simulink model "sampleModel106"  (R2022a)
settings: Solver=VariableStepAuto  StartTime=0.0  StopTime=10.0  RelTol=1e-3
undefined symbols (not defined in the file): DiscIntNeverNeededParam, magnitude, Newton, Raphson
libraries: simulink x379, slpidlib x89
(part 10 of 16)

== system sampleModel106/cfblk79/cfblk7/cfblk11/cfblk12 ==
  cfblk1 : Inport
  cfblk13 : Inport  Port=2
  cfblk14 : Inport  Port=3
  cfblk10 : Signum
  cfblk11 : Constant  Value=[417220800.929518]  SampleTime=1
  cfblk12 : Constant  Value=[-589398286.856220]  SampleTime=1
  cfblk3 : simulink/Discrete/Transfer Fcn First Order  PoleZ=0.95  ICPrevOutput=0.0  DoSatur=off
  cfblk4 : simulink/Discrete/Tapped Delay  vinit=0.0  samptime=-1  NumDelays=1  DelayOrder=Oldest  includeCurrent=off
  cfblk5 : DiscreteStateSpace
  cfblk6 : DiscreteTransferFcn  SampleTime=1
  cfblk7 : Delay  SampleTime=1
  cfblk8 : Sum  Inputs=|++
  cfblk9 : Polyval  Coefs=[ +2.081618890e-019, -1.441693666e-014, +4.719686976e-010, -8.536869453e-006, +1.621573104e-001, -8.087801117e+001 ]
  cfblk2 : Outport
  wires:
  cfblk6/1 -> cfblk5/1
  cfblk5/1 -> cfblk3/1
  cfblk3/1 -> cfblk4/1
  cfblk14/1 -> cfblk7/1
  cfblk13/1 -> cfblk9/1
  cfblk11/1 -> cfblk10/1
  cfblk10/1 -> cfblk6/1
  cfblk8/1 -> cfblk2/1
  cfblk7/1 -> cfblk8/1
  cfblk1/1 -> cfblk8/2

== system sampleModel106/cfblk79/cfblk7/cfblk11/cfblk9 ==
  cfblk1 : Inport
  cfblk11 : Inport  Port=2
  cfblk12 : Inport  Port=3
  cfblk10 : Constant  Value=[-693543349.036448]  SampleTime=1
  cfblk3 : DotProduct  OutDataTypeStr=Inherit: Inherit via internal rule
  cfblk4 : Gain  Gain=[456492011.111705]
  cfblk5 : Rounding
  cfblk6 : Squeeze
  cfblk7 : DotProduct  OutDataTypeStr=Inherit: Inherit via internal rule
  cfblk8 : Signum
  cfblk9 : Constant  Value=[-488837206.320913]  SampleTime=1
  cfblk2 : Outport
  cfblk13 : Outport  Port=2
  cfblk14 : Outport  Port=3
  wires:
  cfblk4/1 -> cfblk14/1
  cfblk5/1 -> cfblk8/1
  cfblk11/1 -> cfblk7/1
  cfblk9/1 -> cfblk5/1
  cfblk10/1 -> cfblk6/1
  cfblk3/1 -> cfblk2/1
  cfblk12/1 -> cfblk7/2
  cfblk6/1 -> cfblk3/1
  cfblk1/1 -> cfblk4/1
  cfblk7/1 -> cfblk13/1
  cfblk8/1 -> cfblk3/2

== system sampleModel106/cfblk79/cfblk7/cfblk12/cfblk11 ==
  cfblk1 : Inport
  cfblk9 : Inport  Port=2
  cfblk3 : simulink/Discrete/Transfer Fcn Real Zero  ZeroZ=0.75  ICPrevInput=0.0  DoSatur=off
      settings: SourceProductBaseCode=SL
  cfblk4 : simulink/Math Operations/MinMax Running Resettable  Function=min  vinit=0.0
  cfblk5 : Sqrt  Operator=rSqrt  AlgorithmType=Newton-Raphson
  cfblk6 : Math  Operator=hermitian
  cfblk7 : UnaryMinus
  cfblk8 : Constant  Value=[197231009.241030]  SampleTime=1
  cfblk2 : Outport
  wires:
  cfblk8/1 -> cfblk7/1
  cfblk1/1 -> cfblk6/1
  cfblk6/1 -> cfblk3/1
  cfblk4/1 -> cfblk2/1
  cfblk3/1 -> cfblk5/1
  cfblk5/1 -> cfblk4/1
  cfblk9/1 -> cfblk4/2

== system sampleModel106/cfblk79/cfblk7/cfblk12/cfblk12 ==
  cfblk1 : Inport
  cfblk10 : Polyval  Coefs=[ +2.081618890e-019, -1.441693666e-014, +4.719686976e-010, -8.536869453e-006, +1.621573104e-001, -8.087801117e+001 ]
  cfblk11 : Constant  Value=[-737910004.264372]  SampleTime=1
  cfblk12 : Constant  Value=[702082945.939267]  SampleTime=1
  cfblk13 : Constant  Value=[-981193615.725488]  SampleTime=1
  cfblk14 : Constant  Value=[-728228126.014809]  SampleTime=1
  cfblk15 : Constant  Value=[-356449572.036937]  SampleTime=1
  cfblk18 : Delay  SampleTime=1
  cfblk3 : DiscreteTransferFcn  SampleTime=1
  cfblk4 : Delay  DelayLengthSource=Input port  SampleTime=1
      settings: InputPortMap=u0,p1
  cfblk5 : UnitDelay  HasFrameUpgradeWarning=on
  cfblk6 : Product
  cfblk7 : Sqrt
  cfblk8 : Rounding
  cfblk9 : Gain  Gain=[623761261.105977]
  cfblk2 : Outport
  cfblk16 : Outport  Port=2
  cfblk17 : Outport  Port=3
  wires:
  cfblk8/1 -> cfblk10/1
  cfblk3/1 -> cfblk6/1
  cfblk15/1 -> cfblk4/1
  cfblk7/1 -> cfblk9/1
  cfblk4/1 -> cfblk16/1
  cfblk9/1 -> cfblk8/1
  cfblk14/1 -> cfblk2/1
  cfblk10/1 -> cfblk5/1
  cfblk13/1 -> cfblk6/2
  cfblk11/1 -> cfblk7/1
  cfblk1/1 -> cfblk4/2
  cfblk5/1 -> cfblk17/1
  cfblk6/1 -> cfblk18/1
  cfblk18/1 -> cfblk3/1

== system sampleModel106/cfblk79/cfblk7/cfblk12/cfblk13 ==
  cfblk1 : Inport
  cfblk10 : Inport  Port=2
  cfblk3 : DiscreteStateSpace
  cfblk4 : DiscreteIntegrator  ICPrevOutput=DiscIntNeverNeededParam  ICPrevScaledInput=DiscIntNeverNeededParam
  cfblk5 : simulink/Discrete/Transfer Fcn Real Zero  ZeroZ=0.75  ICPrevInput=0.0  DoSatur=off
      settings: SourceProductBaseCode=SL
  cfblk6 : Delay  DelayLengthSource=Input port  SampleTime=1
      settings: InputPortMap=u0,p1
  cfblk7 : Sqrt
  cfblk8 : Assignment  DiagnosticForDimensions=Warning  IndexOptions=Index vector (dialog)  Indices=1  OutputSizes=1
  cfblk9 : Sum  Inputs=+
  cfblk2 : Outport
  cfblk11 : Outport  Port=2
  cfblk12 : Outport  Port=3
  wires:
  cfblk6/1 -> cfblk11/1
  cfblk10/1 -> cfblk9/1
  cfblk8/1 -> cfblk5/1
  cfblk7/1 -> cfblk12/1, cfblk3/1, cfblk6/1
  cfblk3/1 -> cfblk8/1
  cfblk9/1 -> cfblk4/1
  cfblk1/1 -> cfblk7/1
  cfblk4/1 -> cfblk8/2, cfblk6/2
  cfblk5/1 -> cfblk2/1

== system sampleModel106/cfblk79/cfblk7/cfblk12/cfblk14 ==
  cfblk1 : Inport
  cfblk12 : Inport  Port=2
  cfblk13 : Inport  Port=3
  cfblk10 : Constant  Value=[-847782743.704588]  SampleTime=1
  cfblk11 : Constant  Value=[54410108.640307]  SampleTime=1
  cfblk17 : Delay  SampleTime=1
  cfblk3 : Product  Inputs=**
  cfblk4 : Sin  TimeSource=Use external signal  SampleTime=0
  cfblk5 : Sqrt  Operator=rSqrt  AlgorithmType=Newton-Raphson
  cfblk6 : Rounding
  cfblk7 : MinMax  Function=max
  cfblk8 : MinMax  Function=max
  cfblk9 : Sum  Inputs=+-
  cfblk2 : Outport
  cfblk14 : Outport  Port=2
  cfblk15 : Outport  Port=3
  cfblk16 : Outport  Port=4
  wires:
  cfblk12/1 -> cfblk15/1
  cfblk9/1 -> cfblk8/1
  cfblk1/1 -> cfblk2/1
  cfblk5/1 -> cfblk4/1
  cfblk10/1 -> cfblk6/1, cfblk7/1
  cfblk6/1 -> cfblk14/1
  cfblk13/1 -> cfblk5/1
  cfblk7/1 -> cfblk16/1
  cfblk4/1 -> cfblk3/1
  cfblk11/1 -> cfblk3/2
  cfblk3/1 -> cfblk9/2
  cfblk8/1 -> cfblk17/1
  cfblk17/1 -> cfblk9/1

== system sampleModel106/cfblk79/cfblk7/cfblk13/cfblk10 ==
  cfblk1 : Inport
  cfblk8 : Inport  Port=2
  cfblk9 : Inport  Port=3
  Action Port : ActionPort  ActionPortLabel=else
  cfblk10 : Delay
  cfblk3 : Delay  DelayLengthSource=Input port
      settings: InputPortMap=u0,p1
  cfblk4 : slpidlib/PID Controller  Controller=PID  Form=Parallel  TimeDomain=Discrete-time  UseExternalTs=off  SampleTime=-1  IntegratorMethod=Forward Euler  FilterMethod=Forward Euler  ControllerParametersSource=internal  P=1  I=1  UseKiTs=off  D=0  N=100  UseFilter=on  TunerSelectOption=Transfer Function Based (PID Tuner App)  InitialConditionSource=internal  InitialConditionForIntegrator=0  InitialConditionForFilter=0  DifferentiatorICPrevScaledInput=0  ExternalReset=none  TrackingMode=off  Kt=1  LimitOutput=off  SatLimitsSource=internal  UpperSaturationLimit=inf  LowerSaturationLimit=-inf  LinearizeAsGain=off  AntiWindupMode=none  Kb=1  POutMin=[]  POutMax=[]  IOutMin=[]  IOutMax=[]  DOutMin=[]  DOutMax=[]  NOutMin=[]  NOutMax=[]  SumOutMin=[]  SumOutMax=[]  SaturationOutMin=[]  SaturationOutMax=[]  PParamMin=[]  PParamMax=[]  IParamMin=[]  IParamMax=[]  DParamMin=[]  DParamMax=[]  NParamMin=[]  NParamMax=[]  KbParamMin=[]  KbParamMax=[]  KtParamMin=[]  KtParamMax=[]  KbOutMin=[]  KbOutMax=[]  KtOutMin=[]  KtOutMax=[]  IntegratorOutMin=[]  IntegratorOutMax=[]  FilterOutMin=[]  FilterOutMax=[]  SumI1OutMin=[]  SumI1OutMax=[]  SumI2OutMin=[]  SumI2OutMax=[]  SumI3OutMin=[]  SumI3OutMax=[]  SumI4OutMin=[]  SumI4OutMax=[]  SumDOutMin=[]  SumDOutMax=[]  DifferentiatorOutMin=[]  DifferentiatorOutMax=[]  FilterDiffOutCoefMin=[]  FilterDiffOutCoefMax=[]  ReciprocalOutMin=[]  ReciprocalOutMax=[]  SumDenOutMin=[]  SumDenOutMax=[]  SumNumOutMin=[]  SumNumOutMax=[]  DivideOutMin=[]  DivideOutMax=[]  UdiffTsProdOutMin=[]  UdiffTsProdOutMax=[]  NTsProdOutMin=[]  NTsProdOutMax=[]  UintegralTsProdOutMin=[]  UintegralTsProdOutMax=[]  UngainTsProdOutMin=[]  UngainTsProdOutMax=[]  IntegratorContinuousStateAttributes=''  IntegratorStateMustResolveToSignalObject=off  IntegratorRTWStateStorageClass=Auto  FilterContinuousStateAttributes=''  FilterStateMustResolveToSignalObject=off  FilterRTWStateStorageClass=Auto  ParallelPVariant=InternalParameters  IdealPVariant=Disabled  IVariant=InternalParameters  DVariant=InternalParameters  IntegratorVariant=Discrete  SatVariant=Disabled  AWVariant=Passthrough  PCopyVariant=Disabled  TRVariant=Disabled  FdbkBlocksVariant=Forward  IdealPFdbkVariant=Disabled  SatFdbkVariant=Disabled  DerivativeFilterVariant=ForwardEulerFilter  NVariant=InternalParameters  NCopyVariant=Disabled  FilterICVariant=InternalICsFilter  IntegratorICVariant=InternalICs  ExternalResetVariant=Disabled  TRSumVariant=Passthrough  SumFdbkVariant=Disabled  SumVariant=Sum_PID  TsampFilterVariant=InternalTs  TsampNgainVariant=Passthrough  TsampIntegralVariant=Passthrough  ExternalSaturationOutDataTypeStr=Inherit: Same as second input  aMode=0
  cfblk5 : Product  Inputs=*
  cfblk6 : PermuteDimensions
  cfblk7 : Sum  Inputs=|++
  cfblk2 : Outport
  wires:
  cfblk8/1 -> cfblk6/1
  cfblk3/1 -> cfblk7/2
  cfblk7/1 -> cfblk5/1
  cfblk9/1 -> cfblk3/1
  cfblk5/1 -> cfblk4/1
  cfblk1/1 -> cfblk3/2
  cfblk6/1 -> cfblk2/1
  cfblk4/1 -> cfblk10/1
  cfblk10/1 -> cfblk7/1

== system sampleModel106/cfblk79/cfblk7/cfblk13/cfblk6 ==
  cfblk1 : Inport
  cfblk6 : Inport  Port=2
  cfblk3 : DiscreteZeroPole  Poles=[0 0.5]  Gain=1
  cfblk4 : simulink/Math Operations/MinMax Running Resettable  Function=min  vinit=0.0
  cfblk5 : Constant  Value=[107048093.151828]  SampleTime=1
  cfblk2 : Outport
  cfblk7 : Outport  Port=2
  wires:
  cfblk5/1 -> cfblk4/1
  cfblk6/1 -> cfblk4/2
  cfblk4/1 -> cfblk7/1, cfblk3/1
  cfblk1/1 -> cfblk2/1

== system sampleModel106/cfblk79/cfblk7/cfblk13/cfblk7 ==
  cfblk1 : Inport
  cfblk11 : Inport  Port=2
  cfblk10 : Constant  Value=[433998706.675589]  SampleTime=1
  cfblk3 : simulink/Discrete/Transfer Fcn First Order  PoleZ=0.95  ICPrevOutput=0.0  DoSatur=off
  cfblk4 : PermuteDimensions
  cfblk5 : Bias  Bias=[753493053.405927]  SaturateOnIntegerOverflow=off
  cfblk6 : Sum  Inputs=+-
  cfblk7 : Sum  Inputs=+
  cfblk8 : Bias  Bias=[552868234.921718]  SaturateOnIntegerOverflow=off
  cfblk9 : Rounding
  cfblk2 : Outport
  cfblk12 : Outport  Port=2
  cfblk13 : Outport  Port=3
  cfblk14 : Outport  Port=4
  wires:
  cfblk1/1 -> cfblk3/1
  cfblk4/1 -> cfblk8/1, cfblk7/1
  cfblk10/1 -> cfblk12/1
  cfblk9/1 -> cfblk13/1, cfblk4/1
  cfblk8/1 -> cfblk2/1
  cfblk11/1 -> cfblk9/1
  cfblk3/1 -> cfblk6/1
  cfblk6/1 -> cfblk14/1
  cfblk7/1 -> cfblk5/1
  cfblk5/1 -> cfblk6/2

== system sampleModel106/cfblk79/cfblk7/cfblk13/cfblk9 ==
  cfblk1 : Inport
  cfblk13 : Inport  Port=2
  Action Port : ActionPort  ActionPortLabel=if(u1 >= 0)
  cfblk10 : Squeeze
  cfblk11 : Constant  Value=[917711784.016903]  SampleTime=1
  cfblk12 : Constant  Value=[-45160633.184772]  SampleTime=1
  cfblk3 : slpidlib/PID Controller  Controller=PID  Form=Parallel  TimeDomain=Discrete-time  UseExternalTs=off  SampleTime=-1  IntegratorMethod=Forward Euler  FilterMethod=Forward Euler  ControllerParametersSource=internal  P=1  I=1  UseKiTs=off  D=0  N=100  UseFilter=on  TunerSelectOption=Transfer Function Based (PID Tuner App)  InitialConditionSource=internal  InitialConditionForIntegrator=0  InitialConditionForFilter=0  DifferentiatorICPrevScaledInput=0  ExternalReset=none  TrackingMode=off  Kt=1  LimitOutput=off  SatLimitsSource=internal  UpperSaturationLimit=inf  LowerSaturationLimit=-inf  LinearizeAsGain=off  AntiWindupMode=none  Kb=1  POutMin=[]  POutMax=[]  IOutMin=[]  IOutMax=[]  DOutMin=[]  DOutMax=[]  NOutMin=[]  NOutMax=[]  SumOutMin=[]  SumOutMax=[]  SaturationOutMin=[]  SaturationOutMax=[]  PParamMin=[]  PParamMax=[]  IParamMin=[]  IParamMax=[]  DParamMin=[]  DParamMax=[]  NParamMin=[]  NParamMax=[]  KbParamMin=[]  KbParamMax=[]  KtParamMin=[]  KtParamMax=[]  KbOutMin=[]  KbOutMax=[]  KtOutMin=[]  KtOutMax=[]  IntegratorOutMin=[]  IntegratorOutMax=[]  FilterOutMin=[]  FilterOutMax=[]  SumI1OutMin=[]  SumI1OutMax=[]  SumI2OutMin=[]  SumI2OutMax=[]  SumI3OutMin=[]  SumI3OutMax=[]  SumI4OutMin=[]  SumI4OutMax=[]  SumDOutMin=[]  SumDOutMax=[]  DifferentiatorOutMin=[]  DifferentiatorOutMax=[]  FilterDiffOutCoefMin=[]  FilterDiffOutCoefMax=[]  ReciprocalOutMin=[]  ReciprocalOutMax=[]  SumDenOutMin=[]  SumDenOutMax=[]  SumNumOutMin=[]  SumNumOutMax=[]  DivideOutMin=[]  DivideOutMax=[]  UdiffTsProdOutMin=[]  UdiffTsProdOutMax=[]  NTsProdOutMin=[]  NTsProdOutMax=[]  UintegralTsProdOutMin=[]  UintegralTsProdOutMax=[]  UngainTsProdOutMin=[]  UngainTsProdOutMax=[]  IntegratorContinuousStateAttributes=''  IntegratorStateMustResolveToSignalObject=off  IntegratorRTWStateStorageClass=Auto  FilterContinuousStateAttributes=''  FilterStateMustResolveToSignalObject=off  FilterRTWStateStorageClass=Auto  ParallelPVariant=InternalParameters  IdealPVariant=Disabled  IVariant=InternalParameters  DVariant=InternalParameters  IntegratorVariant=Discrete  SatVariant=Disabled  AWVariant=Passthrough  PCopyVariant=Disabled  TRVariant=Disabled  FdbkBlocksVariant=Forward  IdealPFdbkVariant=Disabled  SatFdbkVariant=Disabled  DerivativeFilterVariant=ForwardEulerFilter  NVariant=InternalParameters  NCopyVariant=Disabled  FilterICVariant=InternalICsFilter  IntegratorICVariant=InternalICs  ExternalResetVariant=Disabled  TRSumVariant=Passthrough  SumFdbkVariant=Disabled  SumVariant=Sum_PID  TsampFilterVariant=InternalTs  TsampNgainVariant=Passthrough  TsampIntegralVariant=Passthrough  ExternalSaturationOutDataTypeStr=Inherit: Same as second input  aMode=0
  cfblk4 : Assignment  DiagnosticForDimensions=Warning  IndexOptions=Index vector (dialog)  Indices=1  OutputSizes=1
  cfblk5 : Signum
  cfblk6 : Squeeze
  cfblk7 : Squeeze
  cfblk8 : Reshape
  cfblk9 : Sum  Inputs=+-
  cfblk2 : Outport
  cfblk14 : Outport  Port=2
  cfblk15 : Outport  Port=3
  wires:
  cfblk6/1 -> cfblk7/1
  cfblk9/1 -> cfblk2/1
  cfblk7/1 -> cfblk15/1
  cfblk3/1 -> cfblk5/1
  cfblk5/1 -> cfblk8/1
  cfblk8/1 -> cfblk4/1
  cfblk12/1 -> cfblk14/1
  cfblk4/1 -> cfblk6/1, cfblk9/2
  cfblk13/1 -> cfblk10/1
  cfblk1/1 -> cfblk3/1
  cfblk10/1 -> cfblk9/1
  cfblk11/1 -> cfblk4/2

== system sampleModel106/cfblk79/cfblk8/cfblk10/cfblk7 ==
  cfblk1 : Inport
  cfblk6 : Inport  Port=2
  cfblk7 : Inport  Port=3
  cfblk8 : Inport  Port=4
  cfblk9 : Inport  Port=5
  cfblk3 : Delay  DelayLengthSource=Input port  SampleTime=1
      settings: InputPortMap=u0,p1
  cfblk4 : Reshape
  cfblk5 : Constant  Value=[890064737.840276]  SampleTime=1
  cfblk2 : Outport
  wires:
  cfblk9/1 -> cfblk2/1
  cfblk4/1 -> cfblk3/1
  cfblk5/1 -> cfblk3/2
  cfblk8/1 -> cfblk4/1

== system sampleModel106/cfblk79/cfblk8/cfblk10/cfblk8 ==
  cfblk1 : Inport
  cfblk9 : Inport  Port=2
  cfblk10 : Inport  Port=3
  cfblk11 : Inport  Port=4
  cfblk12 : Inport  Port=5
  cfblk3 : DiscreteTransferFcn  SampleTime=1
  cfblk4 : Rounding
  cfblk5 : Sqrt
  cfblk6 : Constant  Value=[743549077.213179]  SampleTime=1
  cfblk7 : Constant  Value=[509884695.187006]  SampleTime=1
  cfblk8 : Constant  Value=[233910695.868611]  SampleTime=1
  cfblk2 : Outport
  cfblk13 : Outport  Port=2
  cfblk14 : Outport  Port=3
  wires:
  cfblk11/1 -> cfblk4/1
  cfblk1/1 -> cfblk5/1
  cfblk10/1 -> cfblk14/1
  cfblk8/1 -> cfblk2/1
  cfblk5/1 -> cfblk13/1
  cfblk12/1 -> cfblk3/1

== system sampleModel106/cfblk79/cfblk8/cfblk11/cfblk11 ==
  cfblk1 : Inport
  cfblk12 : Inport  Port=2
  cfblk13 : Inport  Port=3
  cfblk14 : Inport  Port=4
  cfblk15 : Inport  Port=5
  cfblk16 : Inport  Port=6
  cfblk10 : Constant  Value=[847867701.646288]  SampleTime=1
  cfblk11 : Constant  Value=[-637143935.125896]  SampleTime=1
  cfblk3 : Delay  DelayLengthSource=Input port  SampleTime=1
      settings: InputPortMap=u0,p1
  cfblk4 : Polyval  Coefs=[ +2.081618890e-019, -1.441693666e-014, +4.719686976e-010, -8.536869453e-006, +1.621573104e-001, -8.087801117e+001 ]
  cfblk5 : Sum  Inputs=+
  cfblk6 : Trigonometry
  cfblk7 : Sin  TimeSource=Use external signal  SampleTime=0
  cfblk8 : Bias  Bias=[425461441.150961]  SaturateOnIntegerOverflow=off
  cfblk9 : simulink/Math Operations/MinMax Running Resettable  Function=min  vinit=0.0
  cfblk2 : Outport
  wires:
  cfblk14/1 -> cfblk7/1
  cfblk10/1 -> cfblk8/1
  cfblk16/1 -> cfblk6/1
  cfblk4/1 -> cfblk9/1
  cfblk7/1 -> cfblk4/1
  cfblk1/1 -> cfblk9/2
  cfblk5/1 -> cfblk2/1
  cfblk6/1 -> cfblk3/1
  cfblk13/1 -> cfblk3/2
  cfblk8/1 -> cfblk5/1

== system sampleModel106/cfblk79/cfblk8/cfblk11/cfblk12 ==
  cfblk1 : Inport
  cfblk9 : Inport  Port=2
  cfblk12 : Delay  SampleTime=1
  cfblk3 : simulink/Discrete/Transfer Fcn Real Zero  ZeroZ=0.75  ICPrevInput=0.0  DoSatur=off
      settings: SourceProductBaseCode=SL
  cfblk4 : UnitDelay  HasFrameUpgradeWarning=on
  cfblk5 : Rounding
  cfblk6 : Sum  Inputs=+-
  cfblk7 : DotProduct  OutDataTypeStr=Inherit: Inherit via internal rule
  cfblk8 : Constant  Value=[74573973.878207]  SampleTime=1
  cfblk2 : Outport
  cfblk10 : Outport  Port=2
  cfblk11 : Outport  Port=3
  wires:
  cfblk5/1 -> cfblk4/1
  cfblk8/1 -> cfblk11/1
  cfblk4/1 -> cfblk7/1
  cfblk6/1 -> cfblk7/2, cfblk12/1
  cfblk1/1 -> cfblk2/1
  cfblk7/1 -> cfblk10/1
  cfblk3/1 -> cfblk5/1, cfblk6/2
  cfblk9/1 -> cfblk6/1
  cfblk12/1 -> cfblk3/1

== system sampleModel106/cfblk79/cfblk8/cfblk11/cfblk18 ==
  cfblk1 : Inport
  cfblk8 : Inport  Port=2
  Action Port : ActionPort  ActionPortLabel=if(u1 >= 0)
  cfblk3 : simulink/Discrete/Transfer Fcn First Order  PoleZ=0.95  ICPrevOutput=0.0  DoSatur=off
  cfblk4 : UnitDelay  SampleTime=-1  HasFrameUpgradeWarning=on
  cfblk5 : Delay
  cfblk6 : Constant  Value=[961105.655787]  SampleTime=1
  cfblk7 : Constant  Value=[134183387.324209]  SampleTime=1
  cfblk2 : Outport
  wires:
  cfblk4/1 -> cfblk2/1
  cfblk7/1 -> cfblk4/1
  cfblk5/1 -> cfblk3/1
  cfblk6/1 -> cfblk5/1

== system sampleModel106/cfblk79/cfblk8/cfblk11/cfblk19 ==
  cfblk1 : Inport
  cfblk11 : Inport  Port=2
  cfblk12 : Inport  Port=3
  Action Port : ActionPort  ActionPortLabel=else
  cfblk10 : Sqrt
  cfblk16 : Delay
  cfblk3 : DiscreteFilter
  cfblk4 : DiscreteFir
  cfblk5 : Sum  Inputs=+-
  cfblk6 : Sum  Inputs=+-
  cfblk7 : Bias  Bias=[-421978992.975569]  SaturateOnIntegerOverflow=off
  cfblk8 : Squeeze
  cfblk9 : Product  Inputs=*
  cfblk2 : Outport
  cfblk13 : Outport  Port=2
  cfblk14 : Outport  Port=3
  cfblk15 : Outport  Port=4
  wires:
  cfblk11/1 -> cfblk8/1
  cfblk4/1 -> cfblk2/1, cfblk14/1
  cfblk5/1 -> cfblk7/1
  cfblk9/1 -> cfblk6/2
  cfblk6/1 -> cfblk10/1, cfblk5/2
  cfblk12/1 -> cfblk5/1
  cfblk3/1 -> cfblk4/1, cfblk15/1
  cfblk10/1 -> cfblk13/1
  cfblk1/1 -> cfblk9/1
  cfblk8/1 -> cfblk3/1
  cfblk7/1 -> cfblk16/1
  cfblk16/1 -> cfblk6/1

== system sampleModel106/cfblk79/cfblk8/cfblk9/cfblk9 ==
  cfblk1 : Inport
  cfblk7 : Inport  Port=2
  cfblk8 : Inport  Port=3
  cfblk9 : Inport  Port=4
  cfblk3 : DiscreteStateSpace
  cfblk4 : Polyval  Coefs=[ +2.081618890e-019, -1.441693666e-014, +4.719686976e-010, -8.536869453e-006, +1.621573104e-001, -8.087801117e+001 ]
  cfblk5 : Reshape
  cfblk6 : Constant  Value=[572215483.203508]  SampleTime=1
  cfblk2 : Outport
  cfblk10 : Outport  Port=2
  cfblk11 : Outport  Port=3
  wires:
  cfblk8/1 -> cfblk4/1
  cfblk7/1 -> cfblk2/1
  cfblk1/1 -> cfblk3/1
  cfblk5/1 -> cfblk11/1
  cfblk4/1 -> cfblk10/1
  cfblk3/1 -> cfblk5/1

== system sampleModel106/cfblk80/cfblk10/cfblk10/cfblk10 ==
  cfblk1 : Inport
  cfblk6 : Inport  Port=2
  cfblk3 : DiscreteIntegrator  ICPrevOutput=DiscIntNeverNeededParam  ICPrevScaledInput=DiscIntNeverNeededParam
  cfblk4 : simulink/Discrete/Transfer Fcn First Order  PoleZ=0.95  ICPrevOutput=0.0  DoSatur=off
  cfblk5 : simulink/Math Operations/Slider Gain  gain=1  low=0  high=2
  cfblk2 : Outport
  cfblk7 : Outport  Port=2
  wires:
  cfblk1/1 -> cfblk5/1
  cfblk4/1 -> cfblk7/1
  cfblk6/1 -> cfblk4/1
  cfblk5/1 -> cfblk3/1
  cfblk3/1 -> cfblk2/1

== system sampleModel106/cfblk80/cfblk10/cfblk10/cfblk11 ==
  cfblk1 : Inport
  cfblk9 : Inport  Port=2
  cfblk10 : Delay  SampleTime=1
  cfblk3 : Sum  Inputs=--
  cfblk4 : Sqrt  Operator=rSqrt  AlgorithmType=Newton-Raphson
  cfblk5 : simulink/Math Operations/Slider Gain  gain=1  low=0  high=2
  cfblk6 : Constant  Value=[387218485.302088]  SampleTime=1
  cfblk7 : Constant  Value=[-419599135.660851]  SampleTime=1
  cfblk8 : Constant  Value=[-709917624.129009]  SampleTime=1
  cfblk2 : Outport
  wires:
  cfblk3/1 -> cfblk4/1
  cfblk7/1 -> cfblk2/1
  cfblk9/1 -> cfblk3/2
  cfblk8/1 -> cfblk5/1
  cfblk4/1 -> cfblk10/1
  cfblk10/1 -> cfblk3/1

== system sampleModel106/cfblk80/cfblk10/cfblk10/cfblk12 ==
  cfblk1 : Inport
  cfblk6 : Inport  Port=2
  cfblk7 : Inport  Port=3
  cfblk8 : Inport  Port=4
  cfblk3 : DiscreteStateSpace
  cfblk4 : ComplexToMagnitudeAngle
  cfblk5 : Constant  Value=[132792448.593113]  SampleTime=1
  cfblk2 : Outport
  cfblk9 : Outport  Port=2
  wires:
  cfblk5/1 -> cfblk2/1
  cfblk7/1 -> cfblk3/1
  cfblk4/1 -> cfblk9/1
  cfblk1/1 -> cfblk4/1

== system sampleModel106/cfblk80/cfblk10/cfblk10/cfblk9 ==
  cfblk1 : Inport
  cfblk12 : Inport  Port=2
  cfblk13 : Inport  Port=3
  cfblk10 : Constant  Value=[69698120.127665]  SampleTime=1
  cfblk11 : Constant  Value=[-849367431.639594]  SampleTime=1
  cfblk3 : slpidlib/PID Controller  Controller=PID  Form=Parallel  TimeDomain=Discrete-time  UseExternalTs=off  SampleTime=1  IntegratorMethod=Forward Euler  FilterMethod=Forward Euler  ControllerParametersSource=internal  P=1  I=1  UseKiTs=off  D=0  N=100  UseFilter=on  TunerSelectOption=Transfer Function Based (PID Tuner App)  InitialConditionSource=internal  InitialConditionForIntegrator=0  InitialConditionForFilter=0  DifferentiatorICPrevScaledInput=0  ExternalReset=none  TrackingMode=off  Kt=1  LimitOutput=off  SatLimitsSource=internal  UpperSaturationLimit=inf  LowerSaturationLimit=-inf  LinearizeAsGain=off  AntiWindupMode=none  Kb=1  POutMin=[]  POutMax=[]  IOutMin=[]  IOutMax=[]  DOutMin=[]  DOutMax=[]  NOutMin=[]  NOutMax=[]  SumOutMin=[]  SumOutMax=[]  SaturationOutMin=[]  SaturationOutMax=[]  PParamMin=[]  PParamMax=[]  IParamMin=[]  IParamMax=[]  DParamMin=[]  DParamMax=[]  NParamMin=[]  NParamMax=[]  KbParamMin=[]  KbParamMax=[]  KtParamMin=[]  KtParamMax=[]  KbOutMin=[]  KbOutMax=[]  KtOutMin=[]  KtOutMax=[]  IntegratorOutMin=[]  IntegratorOutMax=[]  FilterOutMin=[]  FilterOutMax=[]  SumI1OutMin=[]  SumI1OutMax=[]  SumI2OutMin=[]  SumI2OutMax=[]  SumI3OutMin=[]  SumI3OutMax=[]  SumI4OutMin=[]  SumI4OutMax=[]  SumDOutMin=[]  SumDOutMax=[]  DifferentiatorOutMin=[]  DifferentiatorOutMax=[]  FilterDiffOutCoefMin=[]  FilterDiffOutCoefMax=[]  ReciprocalOutMin=[]  ReciprocalOutMax=[]  SumDenOutMin=[]  SumDenOutMax=[]  SumNumOutMin=[]  SumNumOutMax=[]  DivideOutMin=[]  DivideOutMax=[]  UdiffTsProdOutMin=[]  UdiffTsProdOutMax=[]  NTsProdOutMin=[]  NTsProdOutMax=[]  UintegralTsProdOutMin=[]  UintegralTsProdOutMax=[]  UngainTsProdOutMin=[]  UngainTsProdOutMax=[]  IntegratorContinuousStateAttributes=''  IntegratorStateMustResolveToSignalObject=off  IntegratorRTWStateStorageClass=Auto  FilterContinuousStateAttributes=''  FilterStateMustResolveToSignalObject=off  FilterRTWStateStorageClass=Auto  ParallelPVariant=InternalParameters  IdealPVariant=Disabled  IVariant=InternalParameters  DVariant=InternalParameters  IntegratorVariant=Discrete  SatVariant=Disabled  AWVariant=Passthrough  PCopyVariant=Disabled  TRVariant=Disabled  FdbkBlocksVariant=Forward  IdealPFdbkVariant=Disabled  SatFdbkVariant=Disabled  DerivativeFilterVariant=ForwardEulerFilter  NVariant=InternalParameters  NCopyVariant=Disabled  FilterICVariant=InternalICsFilter  IntegratorICVariant=InternalICs  ExternalResetVariant=Disabled  TRSumVariant=Passthrough  SumFdbkVariant=Disabled  SumVariant=Sum_PID  TsampFilterVariant=InternalTs  TsampNgainVariant=Passthrough  TsampIntegralVariant=Passthrough  ExternalSaturationOutDataTypeStr=Inherit: Same as second input  aMode=0
  cfblk4 : simulink/Discrete/Transfer Fcn First Order  PoleZ=0.95  ICPrevOutput=0.0  DoSatur=off
  cfblk5 : DiscreteFir  SampleTime=1
  cfblk6 : Product
  cfblk7 : Sin  TimeSource=Use external signal  SampleTime=0
  cfblk8 : Gain  Gain=[-430636425.139552]
  cfblk9 : Constant  Value=[941054476.673307]  SampleTime=1
  cfblk2 : Outport
  wires:
  cfblk4/1 -> cfblk5/1
  cfblk10/1 -> cfblk2/1
  cfblk9/1 -> cfblk6/1
  cfblk7/1 -> cfblk4/1
  cfblk6/1 -> cfblk8/1
  cfblk5/1 -> cfblk3/1
  cfblk13/1 -> cfblk6/2
  cfblk8/1 -> cfblk7/1

== system sampleModel106/cfblk80/cfblk10/cfblk11/cfblk10 ==
  cfblk1 : Inport
  cfblk10 : Inport  Port=2
  cfblk3 : slpidlib/PID Controller  Controller=PID  Form=Parallel  TimeDomain=Discrete-time  UseExternalTs=off  SampleTime=1  IntegratorMethod=Forward Euler  FilterMethod=Forward Euler  ControllerParametersSource=internal  P=1  I=1  UseKiTs=off  D=0  N=100  UseFilter=on  TunerSelectOption=Transfer Function Based (PID Tuner App)  InitialConditionSource=internal  InitialConditionForIntegrator=0  InitialConditionForFilter=0  DifferentiatorICPrevScaledInput=0  ExternalReset=none  TrackingMode=off  Kt=1  LimitOutput=off  SatLimitsSource=internal  UpperSaturationLimit=inf  LowerSaturationLimit=-inf  LinearizeAsGain=off  AntiWindupMode=none  Kb=1  POutMin=[]  POutMax=[]  IOutMin=[]  IOutMax=[]  DOutMin=[]  DOutMax=[]  NOutMin=[]  NOutMax=[]  SumOutMin=[]  SumOutMax=[]  SaturationOutMin=[]  SaturationOutMax=[]  PParamMin=[]  PParamMax=[]  IParamMin=[]  IParamMax=[]  DParamMin=[]  DParamMax=[]  NParamMin=[]  NParamMax=[]  KbParamMin=[]  KbParamMax=[]  KtParamMin=[]  KtParamMax=[]  KbOutMin=[]  KbOutMax=[]  KtOutMin=[]  KtOutMax=[]  IntegratorOutMin=[]  IntegratorOutMax=[]  FilterOutMin=[]  FilterOutMax=[]  SumI1OutMin=[]  SumI1OutMax=[]  SumI2OutMin=[]  SumI2OutMax=[]  SumI3OutMin=[]  SumI3OutMax=[]  SumI4OutMin=[]  SumI4OutMax=[]  SumDOutMin=[]  SumDOutMax=[]  DifferentiatorOutMin=[]  DifferentiatorOutMax=[]  FilterDiffOutCoefMin=[]  FilterDiffOutCoefMax=[]  ReciprocalOutMin=[]  ReciprocalOutMax=[]  SumDenOutMin=[]  SumDenOutMax=[]  SumNumOutMin=[]  SumNumOutMax=[]  DivideOutMin=[]  DivideOutMax=[]  UdiffTsProdOutMin=[]  UdiffTsProdOutMax=[]  NTsProdOutMin=[]  NTsProdOutMax=[]  UintegralTsProdOutMin=[]  UintegralTsProdOutMax=[]  UngainTsProdOutMin=[]  UngainTsProdOutMax=[]  IntegratorContinuousStateAttributes=''  IntegratorStateMustResolveToSignalObject=off  IntegratorRTWStateStorageClass=Auto  FilterContinuousStateAttributes=''  FilterStateMustResolveToSignalObject=off  FilterRTWStateStorageClass=Auto  ParallelPVariant=InternalParameters  IdealPVariant=Disabled  IVariant=InternalParameters  DVariant=InternalParameters  IntegratorVariant=Discrete  SatVariant=Disabled  AWVariant=Passthrough  PCopyVariant=Disabled  TRVariant=Disabled  FdbkBlocksVariant=Forward  IdealPFdbkVariant=Disabled  SatFdbkVariant=Disabled  DerivativeFilterVariant=ForwardEulerFilter  NVariant=InternalParameters  NCopyVariant=Disabled  FilterICVariant=InternalICsFilter  IntegratorICVariant=InternalICs  ExternalResetVariant=Disabled  TRSumVariant=Passthrough  SumFdbkVariant=Disabled  SumVariant=Sum_PID  TsampFilterVariant=InternalTs  TsampNgainVariant=Passthrough  TsampIntegralVariant=Passthrough  ExternalSaturationOutDataTypeStr=Inherit: Same as second input  aMode=0
  cfblk4 : DiscreteZeroPole  Poles=[0 0.5]  Gain=1
  cfblk5 : simulink/Discrete/Difference  ICPrevInput=0.0  OutMin=[]  OutMax=[]  OutDataTypeStr=Inherit: Inherit via back propagation  OutDataType=fixdt(1, 16)  OutScaling=2^-10  DoSatur=off
  cfblk6 : Product  Inputs=**
  cfblk7 : Sqrt  Operator=rSqrt  AlgorithmType=Newton-Raphson
  cfblk8 : Constant  Value=[-878471034.084976]  SampleTime=1
  cfblk9 : Constant  Value=[980508287.317108]  SampleTime=1
  cfblk2 : Outport
  cfblk11 : Outport  Port=2
  cfblk12 : Outport  Port=3
  wires:
  cfblk1/1 -> cfblk3/1
  cfblk5/1 -> cfblk4/1
  cfblk4/1 -> cfblk7/1
  cfblk9/1 -> cfblk11/1
  cfblk3/1 -> cfblk2/1
  cfblk8/1 -> cfblk12/1
  cfblk7/1 -> cfblk6/1
  cfblk10/1 -> cfblk5/1, cfblk6/2

== system sampleModel106/cfblk80/cfblk10/cfblk11/cfblk11 ==
  cfblk1 : Inport
  cfblk9 : Inport  Port=2
  cfblk10 : Delay  SampleTime=1
  cfblk3 : DiscreteStateSpace
  cfblk4 : DiscreteIntegrator  ICPrevOutput=DiscIntNeverNeededParam  ICPrevScaledInput=DiscIntNeverNeededParam
  cfblk5 : simulink/Math Operations/Slider Gain  gain=1  low=0  high=2
  cfblk6 : Rounding
  cfblk7 : UnaryMinus
  cfblk8 : Constant  Value=[833066314.757185]  SampleTime=1
  cfblk2 : Outport
  wires:
  cfblk3/1 -> cfblk7/1
  cfblk4/1 -> cfblk5/1
  cfblk9/1 -> cfblk2/1
  cfblk7/1 -> cfblk6/1
  cfblk8/1 -> cfblk3/1
  cfblk5/1 -> cfblk10/1
  cfblk10/1 -> cfblk4/1

== system sampleModel106/cfblk80/cfblk10/cfblk11/cfblk12 ==
  cfblk1 : Inport
  cfblk10 : Inport  Port=2
  cfblk11 : Inport  Port=3
  cfblk12 : Inport  Port=4
  cfblk3 : Product
  cfblk4 : Product  Inputs=*
  cfblk5 : Gain  Gain=[-892362151.792230]
  cfblk6 : Signum
  cfblk7 : Constant  Value=[-936145302.178599]  SampleTime=1
  cfblk8 : Constant  Value=[-860922800.001276]  SampleTime=1
  cfblk9 : Constant  Value=[-857530112.678363]  SampleTime=1
  cfblk2 : Outport
  cfblk13 : Outport  Port=2
  wires:
  cfblk7/1 -> cfblk5/1
  cfblk8/1 -> cfblk6/1
  cfblk4/1 -> cfblk2/1
  cfblk11/1 -> cfblk13/1
  cfblk10/1 -> cfblk3/1
  cfblk9/1 -> cfblk3/2
  cfblk6/1 -> cfblk4/1

== system sampleModel106/cfblk80/cfblk10/cfblk11/cfblk13 ==
  cfblk1 : Inport
  cfblk6 : Inport  Port=2
  cfblk7 : Inport  Port=3
  cfblk8 : Inport  Port=4
  cfblk3 : Sum  Inputs=+-
  cfblk4 : Product  Inputs=**
  cfblk5 : Polyval  Coefs=[ +2.081618890e-019, -1.441693666e-014, +4.719686976e-010, -8.536869453e-006, +1.621573104e-001, -8.087801117e+001 ]
  cfblk2 : Outport
  cfblk9 : Outport  Port=2
  cfblk10 : Outport  Port=3
  cfblk11 : Outport  Port=4
  cfblk12 : Outport  Port=5
  wires:
  cfblk6/1 -> cfblk9/1
  cfblk1/1 -> cfblk11/1
  cfblk4/1 -> cfblk2/1, cfblk3/2
  cfblk7/1 -> cfblk4/1
  cfblk5/1 -> cfblk4/2
  cfblk8/1 -> cfblk5/1, cfblk3/1
  cfblk3/1 -> cfblk12/1, cfblk10/1

== system sampleModel106/cfblk80/cfblk10/cfblk11/cfblk16 ==
  cfblk1 : Inport
  cfblk13 : Inport  Port=2
  Action Port : ActionPort  ActionPortLabel=if(u1 >= 0)
  cfblk10 : ComplexToMagnitudeAngle
  cfblk11 : Rounding
  cfblk12 : Sum  Inputs=+-
  cfblk15 : Delay
  cfblk3 : simulink/Discrete/Tapped Delay  vinit=0.0  samptime=-1  NumDelays=1  DelayOrder=Oldest  includeCurrent=off
  cfblk4 : simulink/Discrete/Difference  ICPrevInput=0.0  OutMin=[]  OutMax=[]  OutDataTypeStr=Inherit: Inherit via back propagation  OutDataType=fixdt(1, 16)  OutScaling=2^-10  DoSatur=off
  cfblk5 : UnitDelay  SampleTime=-1  HasFrameUpgradeWarning=on
  cfblk6 : DiscreteTransferFcn
  cfblk7 : simulink/Discrete/Transfer Fcn Lead or Lag  PoleZ=0.95  ZeroZ=0.75  ICPrevOutput=0.0  ICPrevInput=0.0  DoSatur=off
      settings: SourceProductBaseCode=SL
  cfblk8 : Assignment  DiagnosticForDimensions=Warning  IndexOptions=Index vector (dialog)  Indices=1  OutputSizes=1
  cfblk9 : simulink/Math Operations/MinMax Running Resettable  Function=min  vinit=0.0
  cfblk2 : Outport
  cfblk14 : Outport  Port=2
  wires:
  cfblk5/1 -> cfblk11/1, cfblk4/1
  cfblk6/1 -> cfblk9/1
  cfblk11/1 -> cfblk3/1
  cfblk7/1 -> cfblk6/1
  cfblk13/1 -> cfblk7/1, cfblk5/1
  cfblk3/1 -> cfblk10/1
  cfblk10/1 -> cfblk14/1
  cfblk4/1 -> cfblk12/1
  cfblk10/2 -> cfblk8/1
  cfblk1/1 -> cfblk2/1
  cfblk9/1 -> cfblk12/2
  cfblk8/1 -> cfblk9/2
  cfblk12/1 -> cfblk15/1
  cfblk15/1 -> cfblk8/2

== system sampleModel106/cfblk80/cfblk10/cfblk11/cfblk17 ==
  cfblk1 : Inport
  cfblk11 : Inport  Port=2
  Action Port : ActionPort  ActionPortLabel=else
  cfblk10 : PermuteDimensions
  cfblk13 : Delay
  cfblk3 : MinMax
  cfblk4 : Sum  Inputs=--
  cfblk5 : Abs  SaturateOnIntegerOverflow=off
  cfblk6 : Abs  SaturateOnIntegerOverflow=off
  cfblk7 : Assignment  DiagnosticForDimensions=Warning  IndexOptions=Index vector (dialog)  Indices=1  OutputSizes=1
  cfblk8 : Sum  Inputs=+-
  cfblk9 : Product  Inputs=*
  cfblk2 : Outport
  cfblk12 : Outport  Port=2
  wires:
  cfblk3/1 -> cfblk5/1, cfblk4/2
  cfblk11/1 -> cfblk2/1, cfblk6/1
  cfblk8/1 -> cfblk3/1
  cfblk4/1 -> cfblk9/1
  cfblk5/1 -> cfblk4/1, cfblk7/2
  cfblk9/1 -> cfblk7/1
  cfblk6/1 -> cfblk10/1
  cfblk10/1 -> cfblk12/1
  cfblk1/1 -> cfblk8/2
  cfblk7/1 -> cfblk13/1
  cfblk13/1 -> cfblk8/1

== system sampleModel106/cfblk80/cfblk10/cfblk11/cfblk9 ==
  cfblk1 : Inport
  cfblk7 : Inport  Port=2
  cfblk8 : Inport  Port=3
  cfblk3 : Delay  ShowEnablePort=on  SampleTime=1
      settings: InputPortMap=u0,e6
  cfblk4 : simulink/Discrete/Transfer Fcn Real Zero  ZeroZ=0.75  ICPrevInput=0.0  DoSatur=off
      settings: SourceProductBaseCode=SL
  cfblk5 : Delay  DelayLengthSource=Input port  SampleTime=1
      settings: InputPortMap=u0,p1
  cfblk6 : Constant  Value=[927284177.162936]  SampleTime=1
  cfblk2 : Outport
  cfblk9 : Outport  Port=2
  cfblk10 : Outport  Port=3
  wires:
  cfblk6/1 -> cfblk2/1
  cfblk5/1 -> cfblk9/1
  cfblk3/1 -> cfblk5/1
  cfblk1/1 -> cfblk4/1
  cfblk4/1 -> cfblk10/1
  cfblk8/1 -> cfblk3/1, cfblk3/2
  cfblk7/1 -> cfblk5/2

== system sampleModel106/cfblk80/cfblk10/cfblk12/cfblk9 ==
  cfblk1 : Inport
  cfblk10 : Constant  Value=[512527277.422146]  SampleTime=1
  cfblk3 : simulink/Discrete/Transfer Fcn Lead or Lag  PoleZ=0.95  ZeroZ=0.75  ICPrevOutput=0.0  ICPrevInput=0.0  DoSatur=off
      settings: SourceProductBaseCode=SL
  cfblk4 : Product  Inputs=**
  cfblk5 : Sqrt  Operator=rSqrt  AlgorithmType=Newton-Raphson
  cfblk6 : Polyval  Coefs=[ +2.081618890e-019, -1.441693666e-014, +4.719686976e-010, -8.536869453e-006, +1.621573104e-001, -8.087801117e+001 ]
  cfblk7 : Bias  Bias=[487378908.068754]  SaturateOnIntegerOverflow=off
  cfblk8 : Constant  Value=[932049116.148268]  SampleTime=1
  cfblk9 : Constant  Value=[-785815421.977476]  SampleTime=1
  cfblk2 : Outport
  cfblk11 : Outport  Port=2
  wires:
  cfblk6/1 -> cfblk11/1
  cfblk1/1 -> cfblk5/1
  cfblk10/1 -> cfblk7/1
  cfblk9/1 -> cfblk4/1
  cfblk8/1 -> cfblk3/1
  cfblk5/1 -> cfblk4/2
  cfblk7/1 -> cfblk2/1
  cfblk4/1 -> cfblk6/1

== system sampleModel106/cfblk80/cfblk10/cfblk16/cfblk6 ==
  cfblk1 : Inport
  cfblk7 : Inport  Port=2
  cfblk8 : Inport  Port=3
  cfblk9 : Inport  Port=4
  cfblk10 : Inport  Port=5
  cfblk3 : Delay  ShowEnablePort=on
      settings: InputPortMap=u0,e6
  cfblk4 : simulink/Math Operations/Slider Gain  gain=1  low=0  high=2
  cfblk5 : Sum  Inputs=+
  cfblk6 : Constant  Value=[-167810608.577483]  SampleTime=1
  cfblk2 : Outport
  cfblk11 : Outport  Port=2
  wires:
  cfblk6/1 -> cfblk5/1
  cfblk3/1 -> cfblk4/1
  cfblk5/1 -> cfblk11/1
  cfblk10/1 -> cfblk3/1
  cfblk7/1 -> cfblk3/2
  cfblk1/1 -> cfblk2/1

== system sampleModel106/cfblk80/cfblk10/cfblk17/cfblk13 ==
  cfblk1 : Inport
  cfblk14 : Inport  Port=2
  cfblk10 : ComplexToRealImag
  cfblk11 : Constant  Value=[934020453.420381]  SampleTime=1
  cfblk12 : Constant  Value=[-69351678.848029]  SampleTime=1
  cfblk13 : Constant  Value=[-137099880.954140]  SampleTime=1
  cfblk3 : DiscreteStateSpace  SampleTime=-1
  cfblk4 : slpidlib/PID Controller  Controller=PID  Form=Parallel  TimeDomain=Discrete-time  UseExternalTs=off  SampleTime=-1  IntegratorMethod=Forward Euler  FilterMethod=Forward Euler  ControllerParametersSource=internal  P=1  I=1  UseKiTs=off  D=0  N=100  UseFilter=on  TunerSelectOption=Transfer Function Based (PID Tuner App)  InitialConditionSource=internal  InitialConditionForIntegrator=0  InitialConditionForFilter=0  DifferentiatorICPrevScaledInput=0  ExternalReset=none  TrackingMode=off  Kt=1  LimitOutput=off  SatLimitsSource=internal  UpperSaturationLimit=inf  LowerSaturationLimit=-inf  LinearizeAsGain=off  AntiWindupMode=none  Kb=1  POutMin=[]  POutMax=[]  IOutMin=[]  IOutMax=[]  DOutMin=[]  DOutMax=[]  NOutMin=[]  NOutMax=[]  SumOutMin=[]  SumOutMax=[]  SaturationOutMin=[]  SaturationOutMax=[]  PParamMin=[]  PParamMax=[]  IParamMin=[]  IParamMax=[]  DParamMin=[]  DParamMax=[]  NParamMin=[]  NParamMax=[]  KbParamMin=[]  KbParamMax=[]  KtParamMin=[]  KtParamMax=[]  KbOutMin=[]  KbOutMax=[]  KtOutMin=[]  KtOutMax=[]  IntegratorOutMin=[]  IntegratorOutMax=[]  FilterOutMin=[]  FilterOutMax=[]  SumI1OutMin=[]  SumI1OutMax=[]  SumI2OutMin=[]  SumI2OutMax=[]  SumI3OutMin=[]  SumI3OutMax=[]  SumI4OutMin=[]  SumI4OutMax=[]  SumDOutMin=[]  SumDOutMax=[]  DifferentiatorOutMin=[]  DifferentiatorOutMax=[]  FilterDiffOutCoefMin=[]  FilterDiffOutCoefMax=[]  ReciprocalOutMin=[]  ReciprocalOutMax=[]  SumDenOutMin=[]  SumDenOutMax=[]  SumNumOutMin=[]  SumNumOutMax=[]  DivideOutMin=[]  DivideOutMax=[]  UdiffTsProdOutMin=[]  UdiffTsProdOutMax=[]  NTsProdOutMin=[]  NTsProdOutMax=[]  UintegralTsProdOutMin=[]  UintegralTsProdOutMax=[]  UngainTsProdOutMin=[]  UngainTsProdOutMax=[]  IntegratorContinuousStateAttributes=''  IntegratorStateMustResolveToSignalObject=off  IntegratorRTWStateStorageClass=Auto  FilterContinuousStateAttributes=''  FilterStateMustResolveToSignalObject=off  FilterRTWStateStorageClass=Auto  ParallelPVariant=InternalParameters  IdealPVariant=Disabled  IVariant=InternalParameters  DVariant=InternalParameters  IntegratorVariant=Discrete  SatVariant=Disabled  AWVariant=Passthrough  PCopyVariant=Disabled  TRVariant=Disabled  FdbkBlocksVariant=Forward  IdealPFdbkVariant=Disabled  SatFdbkVariant=Disabled  DerivativeFilterVariant=ForwardEulerFilter  NVariant=InternalParameters  NCopyVariant=Disabled  FilterICVariant=InternalICsFilter  IntegratorICVariant=InternalICs  ExternalResetVariant=Disabled  TRSumVariant=Passthrough  SumFdbkVariant=Disabled  SumVariant=Sum_PID  TsampFilterVariant=InternalTs  TsampNgainVariant=Passthrough  TsampIntegralVariant=Passthrough  ExternalSaturationOutDataTypeStr=Inherit: Same as second input  aMode=0
  cfblk5 : simulink/Discrete/Tapped Delay  vinit=0.0  samptime=-1  NumDelays=1  DelayOrder=Oldest  includeCurrent=off
  cfblk6 : Rounding
  cfblk7 : Trigonometry
  cfblk8 : Sum  Inputs=+-
  cfblk9 : ComplexToMagnitudeAngle
  cfblk2 : Outport
  cfblk15 : Outport  Port=2
  wires:
  cfblk6/1 -> cfblk7/1
  cfblk7/1 -> cfblk5/1
  cfblk11/1 -> cfblk3/1
  cfblk5/1 -> cfblk9/1
  cfblk4/1 -> cfblk15/1
  cfblk14/1 -> cfblk8/1
  cfblk1/1 -> cfblk10/1
  cfblk12/1 -> cfblk8/2
  cfblk13/1 -> cfblk4/1
  cfblk3/1 -> cfblk6/1
  cfblk8/1 -> cfblk2/1

== system sampleModel106/cfblk80/cfblk10/cfblk17/cfblk14 ==
  cfblk1 : Inport
  cfblk8 : Inport  Port=2
  cfblk9 : Inport  Port=3
  cfblk10 : Inport  Port=4
  cfblk11 : Inport  Port=5
  cfblk12 : Inport  Port=6
  cfblk3 : UnitDelay  SampleTime=-1  HasFrameUpgradeWarning=on
  cfblk4 : Delay
  cfblk5 : Abs  SaturateOnIntegerOverflow=off
  cfblk6 : Squeeze
  cfblk7 : ComplexToRealImag
  cfblk2 : Outport
  cfblk13 : Outport  Port=2
  wires:
  cfblk7/1 -> cfblk13/1
  cfblk9/1 -> cfblk7/1
  cfblk12/1 -> cfblk3/1
  cfblk11/1 -> cfblk5/1
  cfblk3/1 -> cfblk2/1
  cfblk6/1 -> cfblk4/1
  cfblk1/1 -> cfblk6/1

== system sampleModel106/cfblk80/cfblk10/cfblk17/cfblk15 ==
  cfblk1 : Inport
  cfblk9 : Inport  Port=2
  cfblk10 : Inport  Port=3
  cfblk11 : Delay
  cfblk3 : simulink/Discrete/Transfer Fcn Real Zero  ZeroZ=0.75  ICPrevInput=0.0  DoSatur=off
      settings: SourceProductBaseCode=SL
  cfblk4 : Sum  Inputs=+
  cfblk5 : Sqrt
  cfblk6 : Product  Inputs=**
  cfblk7 : Sqrt
  cfblk8 : MinMax
  cfblk2 : Outport
  wires:
  cfblk9/1 -> cfblk3/1
  cfblk4/1 -> cfblk6/1
  cfblk6/1 -> cfblk5/1
  cfblk7/1 -> cfblk2/1
  cfblk10/1 -> cfblk8/1
  cfblk1/1 -> cfblk7/1
  cfblk3/1 -> cfblk4/1
  cfblk5/1 -> cfblk11/1
  cfblk11/1 -> cfblk6/2

== system sampleModel106/cfblk80/cfblk10/cfblk7/cfblk11 ==
  cfblk1 : Inport
  Action Port : ActionPort  ActionPortLabel=if(u1 >= 0)
  cfblk10 : Constant  Value=[229463370.023700]  SampleTime=1
  cfblk11 : Constant  Value=[482450445.305877]  SampleTime=1
  cfblk13 : Delay
  cfblk3 : simulink/Discrete/Difference  ICPrevInput=0.0  OutMin=[]  OutMax=[]  OutDataTypeStr=Inherit: Inherit via back propagation  OutDataType=fixdt(1, 16)  OutScaling=2^-10  DoSatur=off
  cfblk4 : simulink/Discrete/Transfer Fcn Lead or Lag  PoleZ=0.95  ZeroZ=0.75  ICPrevOutput=0.0  ICPrevInput=0.0  DoSatur=off
      settings: SourceProductBaseCode=SL
  cfblk5 : Trigonometry
  cfblk6 : Polyval  Coefs=[ +2.081618890e-019, -1.441693666e-014, +4.719686976e-010, -8.536869453e-006, +1.621573104e-001, -8.087801117e+001 ]
  cfblk7 : Math  Operator=log
  cfblk8 : Sum  Inputs=+-
  cfblk9 : Math  Operator=pow
  cfblk2 : Outport
  cfblk12 : Outport  Port=2
  wires:
  cfblk11/1 -> cfblk4/1
  cfblk10/1 -> cfblk6/1
  cfblk6/1 -> cfblk8/1
  cfblk8/1 -> cfblk2/1
  cfblk4/1 -> cfblk12/1
  cfblk3/1 -> cfblk5/1
  cfblk1/1 -> cfblk9/1
  cfblk7/1 -> cfblk9/2, cfblk13/1
  cfblk5/1 -> cfblk7/1
  cfblk9/1 -> cfblk8/2
  cfblk13/1 -> cfblk3/1

== system sampleModel106/cfblk80/cfblk10/cfblk7/cfblk12 ==
  cfblk1 : Inport
  Action Port : ActionPort  ActionPortLabel=else
  cfblk3 : Math  Operator=mod
  cfblk4 : Product  Inputs=**
  cfblk5 : Constant  Value=[-38439812.553979]  SampleTime=1
  cfblk6 : Constant  Value=[-753511015.414783]  SampleTime=1
  cfblk2 : Outport
  cfblk7 : Outport  Port=2
  wires:
  cfblk6/1 -> cfblk3/1
  cfblk5/1 -> cfblk2/1
  cfblk1/1 -> cfblk4/1, cfblk4/2
  cfblk4/1 -> cfblk3/2
  cfblk3/1 -> cfblk7/1

== system sampleModel106/cfblk80/cfblk10/cfblk7/cfblk7 ==
  cfblk1 : Inport
  cfblk11 : Inport  Port=2
  cfblk10 : Constant  Value=[162740358.929630]  SampleTime=1
  cfblk3 : UnitDelay  HasFrameUpgradeWarning=on
  cfblk4 : Delay  ShowEnablePort=on  SampleTime=1
      settings: InputPortMap=u0,e6
  cfblk5 : Polyval  Coefs=[ +2.081618890e-019, -1.441693666e-014, +4.719686976e-010, -8.536869453e-006, +1.621573104e-001, -8.087801117e+001 ]
  cfblk6 : Constant  Value=[353923936.918538]  SampleTime=1
  cfblk7 : Constant  Value=[608063338.385370]  SampleTime=1
  cfblk8 : Constant  Value=[433153471.595247]  SampleTime=1
  cfblk9 : Constant  Value=[-78079510.726059]  SampleTime=1
  cfblk2 : Outport
  cfblk12 : Outport  Port=2
  wires:
  cfblk6/1 -> cfblk4/1
  cfblk3/1 -> cfblk12/1
  cfblk5/1 -> cfblk2/1
  cfblk1/1 -> cfblk4/2
  cfblk10/1 -> cfblk5/1
  cfblk8/1 -> cfblk3/1

== system sampleModel106/cfblk80/cfblk10/cfblk7/cfblk8 ==
  cfblk1 : Inport
  cfblk10 : Inport  Port=2
  cfblk11 : Inport  Port=3
  cfblk12 : Delay  SampleTime=1
  cfblk3 : slpidlib/PID Controller (2DOF)  Controller=PID  Form=Parallel  TimeDomain=Discrete-time  UseExternalTs=off  SampleTime=1  IntegratorMethod=Forward Euler  FilterMethod=Forward Euler  ControllerParametersSource=internal  P=1  I=1  UseKiTs=off  D=0  N=100  UseFilter=on  b=1  c=1  TunerSelectOption=Transfer Function Based (PID Tuner App)  InitialConditionSource=internal  InitialConditionForIntegrator=0  InitialConditionForFilter=0  DifferentiatorICPrevScaledInput=0  ExternalReset=none  TrackingMode=off  Kt=1  LimitOutput=off  SatLimitsSource=internal  UpperSaturationLimit=inf  LowerSaturationLimit=-inf  LinearizeAsGain=off  AntiWindupMode=none  Kb=1  POutMin=[]  POutMax=[]  IOutMin=[]  IOutMax=[]  DOutMin=[]  DOutMax=[]  NOutMin=[]  NOutMax=[]  bOutMin=[]  bOutMax=[]  cOutMin=[]  cOutMax=[]  SumOutMin=[]  SumOutMax=[]  SaturationOutMin=[]  SaturationOutMax=[]  PParamMin=[]  PParamMax=[]  IParamMin=[]  IParamMax=[]  DParamMin=[]  DParamMax=[]  NParamMin=[]  NParamMax=[]  bParamMin=[]  bParamMax=[]  cParamMin=[]  cParamMax=[]  KbParamMin=[]  KbParamMax=[]  KtParamMin=[]  KtParamMax=[]  KbOutMin=[]  KbOutMax=[]  KtOutMin=[]  KtOutMax=[]  IntegratorOutMin=[]  IntegratorOutMax=[]  FilterOutMin=[]  FilterOutMax=[]  SumI1OutMin=[]  SumI1OutMax=[]  SumI2OutMin=[]  SumI2OutMax=[]  SumI3OutMin=[]  SumI3OutMax=[]  SumI4OutMin=[]  SumI4OutMax=[]  SumDOutMin=[]  SumDOutMax=[]  Sum1OutMin=[]  Sum1OutMax=[]  Sum2OutMin=[]  Sum2OutMax=[]  Sum3OutMin=[]  Sum3OutMax=[]  DifferentiatorOutMin=[]  DifferentiatorOutMax=[]  FilterDiffOutCoefMin=[]  FilterDiffOutCoefMax=[]  ReciprocalOutMin=[]  ReciprocalOutMax=[]  SumDenOutMin=[]  SumDenOutMax=[]  SumNumOutMin=[]  SumNumOutMax=[]  DivideOutMin=[]  DivideOutMax=[]  UdiffTsProdOutMin=[]  UdiffTsProdOutMax=[]  NTsProdOutMin=[]  NTsProdOutMax=[]  UintegralTsProdOutMin=[]  UintegralTsProdOutMax=[]  UngainTsProdOutMin=[]  UngainTsProdOutMax=[]  IntegratorContinuousStateAttributes=''  IntegratorStateMustResolveToSignalObject=off  IntegratorRTWStateStorageClass=Auto  FilterContinuousStateAttributes=''  FilterStateMustResolveToSignalObject=off  FilterRTWStateStorageClass=Auto  ParallelPVariant=InternalParameters  IdealPVariant=Disabled  IVariant=InternalParameters  DVariant=InternalParameters  bVariant=InternalParameters  cVariant=InternalParameters  IntegratorVariant=Discrete  SatVariant=Disabled  AWVariant=Passthrough  PCopyVariant=Disabled  TRVariant=Disabled  FdbkBlocksVariant=Forward  IdealPFdbkVariant=Disabled  SatFdbkVariant=Disabled  DerivativeFilterVariant=ForwardEulerFilter  NVariant=InternalParameters  NCopyVariant=Disabled  FilterICVariant=InternalICsFilter  IntegratorICVariant=InternalICs  ExternalResetVariant=Disabled  TRSumVariant=Passthrough  SumFdbkVariant=Disabled  SumVariant=Sum_PID  TsampFilterVariant=InternalTs  TsampNgainVariant=Passthrough  TsampIntegralVariant=Passthrough  ExternalSaturationOutDataTypeStr=Inherit: Same as second input
      settings: SourceProductBaseCode=SL
  cfblk4 : Squeeze
  cfblk5 : Sum  Inputs=+-
  cfblk6 : Signum
  cfblk7 : PermuteDimensions
  cfblk8 : Constant  Value=[652935742.382168]  SampleTime=1
  cfblk9 : Constant  Value=[549715516.838895]  SampleTime=1
  cfblk2 : Outport
  wires:
  cfblk8/1 -> cfblk5/1
  cfblk10/1 -> cfblk7/1
  cfblk3/1 -> cfblk6/1
  cfblk4/1 -> cfblk2/1
  cfblk6/1 -> cfblk5/2
  cfblk11/1 -> cfblk4/1
  cfblk1/1 -> cfblk3/1
  cfblk5/1 -> cfblk12/1
  cfblk12/1 -> cfblk3/2

== system sampleModel106/cfblk80/cfblk10/cfblk7/cfblk9 ==
  cfblk1 : Inport
  cfblk10 : Rounding
  cfblk11 : Constant  Value=[867221009.773854]  SampleTime=1
  cfblk3 : DiscreteStateSpace
  cfblk4 : simulink/Discrete/Transfer Fcn Real Zero  ZeroZ=0.75  ICPrevInput=0.0  DoSatur=off
      settings: SourceProductBaseCode=SL
  cfblk5 : Squeeze
  cfblk6 : Sum
  cfblk7 : Rounding
  cfblk8 : Squeeze
  cfblk9 : Sum  Inputs=+-
  cfblk2 : Outport
  cfblk12 : Outport  Port=2
  cfblk13 : Outport  Port=3
  cfblk14 : Outport  Port=4
  wires:
  cfblk4/1 -> cfblk5/1
  cfblk10/1 -> cfblk2/1
  cfblk5/1 -> cfblk9/1
  cfblk11/1 -> cfblk7/1
  cfblk8/1 -> cfblk13/1, cfblk3/1
  cfblk3/1 -> cfblk6/1
  cfblk1/1 -> cfblk8/1, cfblk14/1
  cfblk9/1 -> cfblk10/1
  cfblk6/1 -> cfblk4/1, cfblk9/2
  cfblk7/1 -> cfblk6/2, cfblk12/1

== system sampleModel106/cfblk80/cfblk10/cfblk8/cfblk10 ==
  cfblk1 : Inport
  cfblk3 : slpidlib/PID Controller  Controller=PID  Form=Parallel  TimeDomain=Discrete-time  UseExternalTs=off  SampleTime=1  IntegratorMethod=Forward Euler  FilterMethod=Forward Euler  ControllerParametersSource=internal  P=1  I=1  UseKiTs=off  D=0  N=100  UseFilter=on  TunerSelectOption=Transfer Function Based (PID Tuner App)  InitialConditionSource=internal  InitialConditionForIntegrator=0  InitialConditionForFilter=0  DifferentiatorICPrevScaledInput=0  ExternalReset=none  TrackingMode=off  Kt=1  LimitOutput=off  SatLimitsSource=internal  UpperSaturationLimit=inf  LowerSaturationLimit=-inf  LinearizeAsGain=off  AntiWindupMode=none  Kb=1  POutMin=[]  POutMax=[]  IOutMin=[]  IOutMax=[]  DOutMin=[]  DOutMax=[]  NOutMin=[]  NOutMax=[]  SumOutMin=[]  SumOutMax=[]  SaturationOutMin=[]  SaturationOutMax=[]  PParamMin=[]  PParamMax=[]  IParamMin=[]  IParamMax=[]  DParamMin=[]  DParamMax=[]  NParamMin=[]  NParamMax=[]  KbParamMin=[]  KbParamMax=[]  KtParamMin=[]  KtParamMax=[]  KbOutMin=[]  KbOutMax=[]  KtOutMin=[]  KtOutMax=[]  IntegratorOutMin=[]  IntegratorOutMax=[]  FilterOutMin=[]  FilterOutMax=[]  SumI1OutMin=[]  SumI1OutMax=[]  SumI2OutMin=[]  SumI2OutMax=[]  SumI3OutMin=[]  SumI3OutMax=[]  SumI4OutMin=[]  SumI4OutMax=[]  SumDOutMin=[]  SumDOutMax=[]  DifferentiatorOutMin=[]  DifferentiatorOutMax=[]  FilterDiffOutCoefMin=[]  FilterDiffOutCoefMax=[]  ReciprocalOutMin=[]  ReciprocalOutMax=[]  SumDenOutMin=[]  SumDenOutMax=[]  SumNumOutMin=[]  SumNumOutMax=[]  DivideOutMin=[]  DivideOutMax=[]  UdiffTsProdOutMin=[]  UdiffTsProdOutMax=[]  NTsProdOutMin=[]  NTsProdOutMax=[]  UintegralTsProdOutMin=[]  UintegralTsProdOutMax=[]  UngainTsProdOutMin=[]  UngainTsProdOutMax=[]  IntegratorContinuousStateAttributes=''  IntegratorStateMustResolveToSignalObject=off  IntegratorRTWStateStorageClass=Auto  FilterContinuousStateAttributes=''  FilterStateMustResolveToSignalObject=off  FilterRTWStateStorageClass=Auto  ParallelPVariant=InternalParameters  IdealPVariant=Disabled  IVariant=InternalParameters  DVariant=InternalParameters  IntegratorVariant=Discrete  SatVariant=Disabled  AWVariant=Passthrough  PCopyVariant=Disabled  TRVariant=Disabled  FdbkBlocksVariant=Forward  IdealPFdbkVariant=Disabled  SatFdbkVariant=Disabled  DerivativeFilterVariant=ForwardEulerFilter  NVariant=InternalParameters  NCopyVariant=Disabled  FilterICVariant=InternalICsFilter  IntegratorICVariant=InternalICs  ExternalResetVariant=Disabled  TRSumVariant=Passthrough  SumFdbkVariant=Disabled  SumVariant=Sum_PID  TsampFilterVariant=InternalTs  TsampNgainVariant=Passthrough  TsampIntegralVariant=Passthrough  ExternalSaturationOutDataTypeStr=Inherit: Same as second input  aMode=0
  cfblk4 : Product
  cfblk5 : DotProduct  OutDataTypeStr=Inherit: Inherit via internal rule
  cfblk6 : Constant  Value=[-771823005.444604]  SampleTime=1
  cfblk7 : Constant  Value=[-57925706.222643]  SampleTime=1
  cfblk9 : Delay  SampleTime=1
  cfblk2 : Outport
  cfblk8 : Outport  Port=2
  wires:
  cfblk3/1 -> cfblk2/1, cfblk5/2
  cfblk6/1 -> cfblk8/1
  cfblk1/1 -> cfblk4/1
  cfblk4/1 -> cfblk5/1
  cfblk7/1 -> cfblk3/1
  cfblk5/1 -> cfblk9/1
  cfblk9/1 -> cfblk4/2
